simulink model "StateMachinaTesting"  (R2016a)
settings: Solver=VariableStepAuto  StartTime=0.0  StopTime=orbit_length*40  RelTol=1e-3
values from neighbouring files (symbols this model uses):
  A = eye(16,16)    [full_input_list.m]
  B = zeros(16,1)    [full_input_list.m]
  C = blkdiag(eye(3,3),zeros(3,3),eye(10,10))    [full_input_list.m]
  counter = 0    [full_input_list.m]
  deltaT = 0.00001    (= 1e-05)    [full_input_list.m]
  H = C    [full_input_list.m]
  kd = 0.5    [full_input_list.m]    (also in initACS.m = 0.01)
  kp = 1    [full_input_list.m]    (also in initACS.m = 0.01)
  OpModes = [0 0 0]    [full_input_list.m]
  OpTimes = [0 1 2]    [full_input_list.m]
  Q_k = zeros(16,16)    [full_input_list.m]
  R = R_k    [full_input_list.m]
  SeperationTime = 30000    [full_input_list.m]
  sim_start_time = (JD - JD_GPS0) * 24*60*60 - UTC_leap_seconds_wrt_GPS    (= 36000.0287935)    [full_input_list.m]
  st = 1/freq    (= 0.0125)    [full_input_list.m]    (also in initSimulink.m)
  u_k = zeros(16,1)    [full_input_list.m]
  w_k = zeros(16,1)    [full_input_list.m]
  x0 = [0 ... (first row only)    [full_input_list.m]
  Z_k = zeros(16,1)    [full_input_list.m]
undefined symbols (not defined in the file or in its folder): DiscIntNeverNeededParam, Earth, G_igrf, gyro_DCM_BS, H_igrf, I_undeployed, IAU, km, Kschmidt, mag_variance, n, R_mean, sat2, WGS84
libraries: simulink x29, dspmathops x24, aerolibutil x20, aerolibtransform2 x20, vrlib x15, aerolibgravity2 x5, dspinverses x4, SimMainLibrary x3, dspmtrx3 x1, lib_violet_env x1
(part 2 of 4)

== system StateMachinaTesting/Sensors MUXED/Center Cube Sensors ==
  note: TEMPORARY TO CHECK DATA EVALUATION AT LKF LEVEL
      | THIS IS AN ENTIRELY RBF SECTION
  note: r_N is in format:
      | - Lat (N-S) in decimal deg
      | - Long (E-W) in decimal deg
      | - Height in m
  State : Inport
  Add{1,3,5,7} (4 alike) : Sum
  Band-Limited White  Noise3 : simulink/Sources/Band-Limited White Noise  Cov=[1e-5]  Ts=0.1  seed=[23341]
  Band-Limited White Noise1 : simulink/Sources/Band-Limited White Noise  Cov=[0.1]  Ts=st  seed=[23341]
  Band-Limited White Noise5 : simulink/Sources/Band-Limited White Noise  Cov=[0.1]  Ts=0.1  seed=[23341]
  Band-Limited White Noise7 : simulink/Sources/Band-Limited White Noise  Cov=[0.1]  Ts=0.1  seed=[23341]
  Bus Creator2 : BusCreator  Inputs=6
  Bus Selector5 : BusSelector  OutputSignals=r_N,v_N,q_BN,w_BN
  Clock : Clock
  Constant : Constant  Value=sim_start_time
  Create Mag Vector : Subsystem
  Create Sun Vector : Subsystem  AncestorBlock=SimMainLibrary/SideCubeSensors/Create Sun Vector
  Derivative : Derivative
  Display : Display
  Subsystem : Subsystem
  Sum2 : Sum  Inputs=|++
  Sensors : Outport
  wires:
  Add1/1 -> Bus Creator2/1  "accelerometer_1"
  Band-Limited White Noise1/1 -> Add1/1
  Subsystem/1(a_B) -> Add1/2  "a_B"
  Band-Limited White  Noise3/1 -> Add3/1
  State/1 -> Bus Selector5/1
  Bus Creator2/1 -> Sensors/1
  Derivative/1 -> Subsystem/1("a_N ")  "a_N"
  Add7/1 -> Bus Creator2/3  "sun_B"
  Sum2/1 -> Create Sun Vector/2(time), Create Mag Vector/3(time), Bus Creator2/6  "time"
  Add3/1 -> Bus Creator2/2  "w_BN_1"
  Band-Limited White Noise7/1 -> Add7/1
  Create Sun Vector/1(sun_B) -> Add7/2  "sun_B"
  [r_N] -> Bus Creator2/4
  Create Mag Vector/1(mag_B) -> Add5/2
  Add5/1 -> Bus Creator2/5  "magnetometer_1"
  Band-Limited White Noise5/1 -> Add5/1
  [r_N] -> Create Mag Vector/2(r_N)
  Bus Selector5/1 -> [r_N]  "<r_N>"
  Bus Selector5/2 -> Derivative/1  "<v_N>"
  Bus Selector5/3 -> Subsystem/2(q_BN), Create Mag Vector/1(q_BN), Create Sun Vector/1(q_BN)  "<q_BN>"
  Bus Selector5/4 -> Add3/2  "<w_BN>"
  Constant/1 -> Sum2/1, Display/1
  Clock/1 -> Sum2/2

== system StateMachinaTesting/Sun Pointing/Target Quaternion ==
  w_c : Inport
  q4 : Inport  Port=2
  Constant : Constant  Value=pi
  Phi/2 : Trigonometry  Operator=acos
  Product : Product
  Terminator : Terminator
  Trigonometric Function1 : Trigonometry
  Trigonometric Function2 : Trigonometry  Operator=cos
  Vector Concatenate : Concatenate
  q_target : Outport
  wires:
  Vector Concatenate/1 -> q_target/1
  w_c/1 -> Product/1
  Product/1 -> Vector Concatenate/1
  Trigonometric Function1/1 -> Product/2
  Trigonometric Function2/1 -> Vector Concatenate/2
  q4/1 -> Phi/2/1
  Phi/2/1 -> Terminator/1
  Constant/1 -> Trigonometric Function2/1, Trigonometric Function1/1

== system StateMachinaTesting/x_measured1/Lookup Tables ==
  note: r_N is in format:
      | - Lat (N-S) in decimal deg
      | - Long (E-W) in decimal deg
      | - Height in m
  x_pos : Inport
  time : Inport  Port=2
  Demux : Demux  Outputs=3
  ECI Position to LLA : aerolibtransform2/ECI Position to LLA  Commented=on  red=IAU-2000/2006  year=2016  month=September  day=20  hour=0  min=0  sec=0  deltaT=Sec  errorflag=Error  extraparamflag=off  eunits=Metric (MKS)  earthmodel=WGS84  flat=1/298.257223563  eqradius=6378137
      settings: AttributesFormatString=%<red>
  GPS time to Jd sfrom J2000 : Subsystem
  Normalization : dspmathops/Normalization  NormType=2-norm  Bias=1e-10  NormOver=Each column  Dimension=1  outputDataTypeStr=Inherit: Same as product output  outputLastDataTypeStr=Inherit: Same as product output  outputMin=[]  outputMax=[]  accumDataTypeStr=Inherit: Same as product output  accumLastDataTypeStr=Inherit: Same as product output  roundingMode=Floor  overflowMode=off
  "RBF!!!!! " : Constant  Value=2015
  Sun position off of Jd frm J2000 : Subsystem
  Terminator{,1..3} (4 alike) : Terminator
  World Magnetic Model 2015 : aerolibgravity2/World Magnetic Model 2015  Commented=on  units=Metric (MKS)  time_in=on  month=January  day=1  year=2015  action=Error  h_out=on  dec_out=on  inc_out=on  ti_out=on
  B_N : Outport
  V_sun_N : Outport  Port=2
  wires:
  Sun position off of Jd frm J2000/1(Out1) -> Normalization/1
  GPS time to Jd sfrom J2000/1(Out1) -> Sun position off of Jd frm J2000/1(In1)
  Normalization/1 -> V_sun_N/1  "s_hat_N"
  time/1 -> ECI Position to LLA/2, GPS time to Jd sfrom J2000/1(In1)
  "RBF!!!!! "/1 -> World Magnetic Model 2015/4
  ECI Position to LLA/1 -> Demux/1
  x_pos/1 -> ECI Position to LLA/1
  World Magnetic Model 2015/5 -> Terminator3/1
  World Magnetic Model 2015/4 -> Terminator2/1
  World Magnetic Model 2015/3 -> Terminator1/1
  World Magnetic Model 2015/2 -> Terminator/1
  World Magnetic Model 2015/1 -> B_N/1
  Demux/2 -> World Magnetic Model 2015/3
  Demux/1 -> World Magnetic Model 2015/2
  Demux/3 -> World Magnetic Model 2015/1

== system StateMachinaTesting/x_measured1/q_N from Sensors ==
  B_B : Inport
  V_sun_B : Inport  Port=2
  B_N : Inport  Port=3
  V_sun_N : Inport  Port=4
  Cross Product{1..4} (4 alike) : vrlib/Utilities/Cross Product
  Direction Cosine Matrix to Quaternions : aerolibtransform2/Direction Cosine Matrix  to Quaternions
  Normalization{1..4} (4 alike) : dspmathops/Normalization  NormType=2-norm  Bias=1e-10  NormOver=Each column  Dimension=1  outputDataTypeStr=Inherit: Same as product output  outputLastDataTypeStr=Inherit: Same as product output  outputMin=[]  outputMax=[]  accumDataTypeStr=Inherit: Same as product output  accumLastDataTypeStr=Inherit: Same as product output  roundingMode=Floor  overflowMode=off
  Product : Product  Multiplication=Matrix(*)
  Pseudoinverse : dspinverses/Pseudoinverse  wanterr=off
  Vector Concatenate : Concatenate  NumInputs=3  Mode=Multidimensional array  ConcatenateDimension=2
  Vector Concatenate1 : Concatenate  NumInputs=3  Mode=Multidimensional array  ConcatenateDimension=2
  quat From DCM : MATLAB Function  Commented=on  TreatAsAtomicUnit=on
  q_N : Outport
  Q : Outport  Port=2
  wires:
  Vector Concatenate1/1 -> Pseudoinverse/1
  Pseudoinverse/1 -> Product/2
  Product/1 -> Q/1, Direction Cosine Matrix to Quaternions/1
  Vector Concatenate/1 -> Product/1
  Cross Product4/1 -> Vector Concatenate/1  "n_1"
  Normalization3/1 -> Cross Product4/2, Vector Concatenate/3  "n_3"
  Normalization4/1 -> Cross Product4/1, Vector Concatenate/2  "n_2"
  Cross Product2/1 -> Normalization3/1
  B_N/1 -> Normalization4/1, Cross Product2/2
  Cross Product3/1 -> Vector Concatenate1/1  "b_1"
  Normalization1/1 -> Cross Product3/2, Vector Concatenate1/3  "b_3"
  Normalization2/1 -> Cross Product3/1, Vector Concatenate1/2  "b_2"
  Cross Product1/1 -> Normalization1/1
  B_B/1 -> Normalization2/1, Cross Product1/2
  V_sun_B/1 -> Cross Product1/1
  V_sun_N/1 -> Cross Product2/1
  Direction Cosine Matrix to Quaternions/1 -> q_N/1

== system StateMachinaTesting/Flight Controller/Center Cube Controller/Attitude Compensator ==
  note: Commands of 4 burn wires; two for sidecube deploy
      | and two for stabilizing wires
  note: Action Block
      | Notes: This block determines the actions the satellite will execute based on the commands given by ground control/ powerboard.
      | -Possible we end up combining this and the guidance block for simplicity
  SafedOpMode : Inport
  SafedSepBurn : Inport  Port=2
  q2 : Inport  Port=3
  w2 : Inport  Port=4
  Bus Creator : BusCreator  Inputs=2
  Constant : Constant  Value=[ 1 1 1 1 ]
  Deployed Modes (switch)1 : Subsystem
  Merge2 : Merge
  Not Deployed Modes (switch) : Subsystem
  Selector : Selector  InputPortWidth=4  IndexOptions=Index vector (dialog)  Indices=[1]  OutputSizes=1
  Switch Case : SwitchCase  CaseConditions={0,1}  ShowDefaultCase=off
  Terminator : Terminator
  OpMode : Outport
  SepBurn : Outport  Port=2
  Tau1 : Outport  Port=3
  wires:
  SafedOpMode/1 -> [OpMode], OpMode/1
  Merge2/1 -> Tau1/1
  Not Deployed Modes (switch)/1(Out1) -> Merge2/1
  q2/1 -> [Quaternion]
  w2/1 -> [SpinRate]
  [Quaternion] -> Not Deployed Modes (switch)/2(q_BN)
  [SpinRate] -> Not Deployed Modes (switch)/3(w_BN)
  [Quaternion] -> Deployed Modes (switch)1/2(q1)
  [SpinRate] -> Deployed Modes (switch)1/3(w1)
  Deployed Modes (switch)1/1(Out1) -> Merge2/2
  [SafedSepBurn] -> Selector/1
  Constant/1 -> SepBurn/1, [SafedSepBurn]
  Switch Case/1 -> Not Deployed Modes (switch)/Action  "SafedSepBurn"
  Switch Case/2 -> Deployed Modes (switch)1/Action  "SafedSepBurn"
  [OpMode] -> Bus Creator/1
  Bus Creator/1 -> Not Deployed Modes (switch)/1(Mode and BurnCmd), Deployed Modes (switch)1/1(Mode and BurnCmd)
  [SafedSepBurn] -> Bus Creator/2  "SeperationCommand"
  SafedSepBurn/1 -> Terminator/1
  Selector/1 -> Switch Case/1

== system StateMachinaTesting/Flight Controller/Center Cube Controller/Motor Control Placeholder ==
  note: Tether Control Sybsystem
      | When the spin rate of the CubeSat reaches
      | 6rpm, the tether will unreel a set amount
  spin rate : Inport
  SafedOpMode : Inport  Port=2
  If : If  NumInputs=2  IfExpression=u1 > 5 & u2 > 0
  Math Function : Math  Operator=square  SaturateOnIntegerOverflow=on
  Merge : Merge
  Mux : Mux  Inputs=2
  Spinning fast : Subsystem  TreatAsAtomicUnit=on
  Spinning slow : Subsystem  TreatAsAtomicUnit=on
  Sqrt : Sqrt  SaturateOnIntegerOverflow=on
  Sum of Elements : Sum  Inputs=+
  motor cmd : Outport
  wires:
  Math Function/1 -> Sum of Elements/1
  Sum of Elements/1 -> Sqrt/1
  spin rate/1 -> Math Function/1
  Sqrt/1 -> If/1
  Spinning fast/1(Out1) -> Merge/1
  Spinning slow/1(Out1) -> Merge/2
  If/1 -> Spinning fast/Action
  If/2 -> Spinning slow/Action
  SafedOpMode/1 -> If/2
  Mux/1 -> motor cmd/1
  Merge/1 -> Mux/2, Mux/1

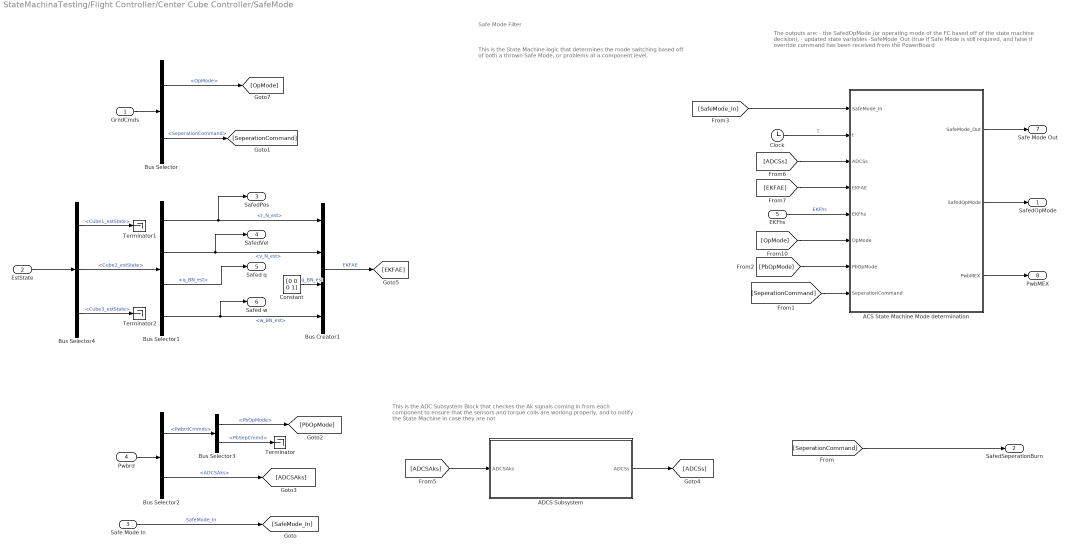
== system StateMachinaTesting/Flight Controller/Center Cube Controller/SafeMode ==
  note: This is the State Machine logic that determines the mode switching based off of both a thrown Safe Mode, or problems at a component level.
  note: Safe Mode Filter
  note: The outputs are:
      | - the SafedOpMode (or operating mode of the FC based off of the state machine decision),
      | - updated state variables
      | -SafeMode_Out (true if Safe Mode is still required, and false if override command has been received from the PowerBoard
  note: This is the ADC Subsystem Block that checkes the Ak signals coming in from each component to ensure that the sensors and torque coils are working properly, and to notify the State Machine in case they are not
  GrndCmds : Inport
  EstState : Inport  Port=2
  Safe Mode In : Inport  Port=3
  Pwbrd : Inport  Port=4
  "EKFhs " : Inport  Port=5
  ACS State Machine Mode determination : MATLAB Function  TreatAsAtomicUnit=on
  ADCS Subsystem : Subsystem
  Bus Creator1 : BusCreator  Inputs='r_N_est','v_N_est','q_BN_est','w_BN_est'
  Bus Selector : BusSelector  OutputSignals=OpMode,SeperationCommand
  Bus Selector1 : BusSelector  OutputSignals=r_N_est,v_N_est,q_BN_est,w_BN_est
  Bus Selector2 : BusSelector  OutputSignals=PwbrdCmmds,ADCSAks
  Bus Selector3 : BusSelector  OutputSignals=PbOpMode,PbSepCmmd
  Bus Selector4 : BusSelector  OutputSignals=Cube1_estState,Cube2_estState,Cube3_estState
  Clock : Clock
  Constant : Constant  Value=[0 0 0 1]
  Terminator : Terminator
  Terminator1 : Terminator
  Terminator2 : Terminator
  SafedOpMode : Outport
  SafedSeperationBurn : Outport  Port=2
  SafedPos : Outport  Port=3
  SafedVel : Outport  Port=4
  Safed q : Outport  Port=5
  Safed w : Outport  Port=6
  Safe Mode Out : Outport  Port=7
  PwbMEX : Outport  Port=8
  wires:
  Clock/1 -> ACS State Machine Mode determination/2(t)  "t"
  "EKFhs "/1 -> ACS State Machine Mode determination/5(EKFhs)  "EKFhs"
  [ADCSs] -> ACS State Machine Mode determination/3(ADCSs)
  Bus Selector1/4 -> Safed w/1, Bus Creator1/4  "<w_BN_est>"
  Bus Selector1/3 -> Safed q/1  "<q_BN_est>"
  Bus Selector1/2 -> SafedVel/1, Bus Creator1/2  "<v_N_est>"
  Bus Selector1/1 -> SafedPos/1, Bus Creator1/1  "<r_N_est>"
  EstState/1 -> Bus Selector4/1
  Bus Selector/1 -> [OpMode]  "<OpMode>"
  GrndCmds/1 -> Bus Selector/1
  Safe Mode In/1 -> [SafeMode_In]  "SafeMode_In"
  ACS State Machine Mode determination/1(SafeMode_Out) -> Safe Mode Out/1
  Bus Selector/2 -> [SeperationCommand]  "<SeperationCommand>"
  [SeperationCommand] -> SafedSeperationBurn/1
  [SeperationCommand] -> ACS State Machine Mode determination/8(SeperationCommand)
  Pwbrd/1 -> Bus Selector2/1
  Bus Selector2/2 -> [ADCSAks]  "<ADCSAks>"
  [ADCSAks] -> ADCS Subsystem/1("ADCSAks ")
  Bus Selector2/1 -> Bus Selector3/1  "<PwbrdCmmds>"
  Bus Selector3/1 -> [PbOpMode]  "<PbOpMode>"
  [OpMode] -> ACS State Machine Mode determination/6(OpMode)
  [PbOpMode] -> ACS State Machine Mode determination/7(PbOpMode)
  Bus Creator1/1 -> [EKFAE]  "EKFAE"
  [EKFAE] -> ACS State Machine Mode determination/4(EKFAE)
  ACS State Machine Mode determination/2(SafedOpMode) -> SafedOpMode/1
  ACS State Machine Mode determination/3(PwbMEX) -> PwbMEX/1
  Bus Selector3/2 -> Terminator/1  "<PbSepCmmd>"
  ADCS Subsystem/1("ADCSs ") -> [ADCSs]
  [SafeMode_In] -> ACS State Machine Mode determination/1(SafeMode_In)
  Constant/1 -> Bus Creator1/3  "q_BN_est"
  Bus Selector4/2 -> Bus Selector1/1  "<Cube2_estState>"
  Bus Selector4/1 -> Terminator1/1  "<Cube1_estState>"
  Bus Selector4/3 -> Terminator2/1  "<Cube3_estState>"

== system StateMachinaTesting/Flight Controller/Center Cube Controller/Torque Coil Management ==
  note: Navigation Block
      | This block takes in data from the Actions/guidance block as to the current attitude of the spacecraft, the desired attitude of the spacecraft, and the required torque and outputs the current necessary to be applied to the torque coils as well as the torque currently being applied by the torque coils.
  BurnCmd : Inport
  q_BN : Inport  Port=2
  w : Inport  Port=3
  tau_B : Inport  Port=4
  b_N : Inport  Port=5
  Clock : Clock
  Constant : Constant
  Constant b_N field RBF!!!!!!!!!!!!!!!! SUB IN THE b_N : Constant  Value=[1 1 1]
  Constant1 : Constant
  Counter : Constant  Value=counter
  If : If  NumInputs=2  IfExpression=(u1 > 0)|(u2>5)
  Measurement Predicition : Subsystem
  Merge1 : Merge
  Merge2 : Merge
  No Action : Subsystem  TreatAsAtomicUnit=on
  PD Controller : Subsystem
  Selector : Selector  Commented=on  InputPortWidth=4  IndexOptions=Index vector (dialog)  Indices=[1]  OutputSizes=1
  Terminator : Terminator
  Terminator1 : Terminator
  Terminator3 : Terminator
  Torque Coil Management : Subsystem  TreatAsAtomicUnit=on
  CenterCube_PWM_cmds : Outport
  torque_coils : Outport  Port=2
  wires:
  BurnCmd/1 -> Selector/1
  If/1 -> Torque Coil Management/Action
  Merge1/1 -> CenterCube_PWM_cmds/1
  Merge2/1 -> torque_coils/1
  Torque Coil Management/1(current_coils) -> Merge1/1
  Torque Coil Management/2(torque_coils) -> Merge2/1
  No Action/1(I_coils) -> Merge1/2
  No Action/2(torque_coils) -> Merge2/2
  q_BN/1 -> Torque Coil Management/2(q_BN)
  tau_B/1 -> Torque Coil Management/1(tau_B)
  w/1 -> PD Controller/1(In1)
  PD Controller/1(torque_coils) -> Terminator3/1
  Measurement Predicition/1(predicition) -> Terminator1/1
  Clock/1 -> Torque Coil Management/4(t)
  If/2 -> No Action/Action
  Counter/1 -> If/2
  Constant/1 -> Measurement Predicition/1(GPS_time)
  Constant1/1 -> Measurement Predicition/2(something else)
  Selector/1 -> If/1
  Constant b_N field RBF!!!!!!!!!!!!!!!! SUB IN THE b_N/1 -> Torque Coil Management/3(b_N)
  b_N/1 -> Terminator/1

== system StateMachinaTesting/Flight Controller/CenterCube EKF/Kalman Gain and Estamated State Computation ==
  P_kp : Inport
  x_kp : Inport  Port=2
  Y : Inport  Port=3
  " LU Inverse" : dspinverses/ LU Inverse
  Add1 : Sum
  Add2 : Sum
  Add3 : Sum  Inputs=-+
  H : Constant  Value=H
  H1 : Constant  Value=H
  Math Function : Math  Operator=transpose  SaturateOnIntegerOverflow=on
  Product{,1,3..4,6} (5 alike) : Product  Multiplication=Matrix(*)
  Product2 : Product
  R : Constant  Value=R
  K : Outport
  x_k : Outport  Port=2
  wires:
  H/1 -> Product3/1, Product1/2, Math Function/1
  " LU Inverse"/1 -> Product/2
  Product1/1 -> Product/1
  Math Function/1 -> Product4/2
  Product/1 -> Product2/1, K/1  "Kalman Gain K"
  x_kp/1 -> Add2/1, Product6/2
  Y/1 -> Add3/2
  R/1 -> Add1/2
  Product4/1 -> Add1/1
  Add1/1 -> " LU Inverse"/1
  Product3/1 -> Product4/1
  H1/1 -> Product6/1
  Product6/1 -> Add3/1
  P_kp/1 -> Product3/2, Product1/1
  Add2/1 -> x_k/1
  Add3/1 -> Product2/2
  Product2/1 -> Add2/2

== system StateMachinaTesting/Flight Controller/CenterCube EKF/New State Prediction  ==
  note: LKF
  note: EKF
  P_k-1 : Inport
  x_k-1 : Inport  Port=2
  A_LKF : Subsystem
  Add1 : Sum  Inputs=+++
  Add2 : Sum
  Add3 : Sum
  B : Constant  Value=B
  Math Function : Math  Operator=transpose  SaturateOnIntegerOverflow=on
  Math Function1 : Math  Operator=transpose  SaturateOnIntegerOverflow=on
  Predictions : MATLAB Function  TreatAsAtomicUnit=on
  Product{,1..5} (6 alike) : Product  Multiplication=Matrix(*)
  Q_k : Constant  Value=Q_k
  Q_k1 : Constant  Value=Q_k
  Terminator2 : Terminator
  Terminator3 : Terminator
  u_k : Constant  Value=u_k
  w_k : Constant  Value=w_k
  P_kp : Outport
  "x_kp  " : Outport  Port=2
  wires:
  Product2/1 -> Product3/1
  Math Function/1 -> Product3/2
  Product/1 -> Add1/1
  B/1 -> Product1/1
  Product1/1 -> Add1/2
  u_k/1 -> Product1/2
  w_k/1 -> Add1/3
  Q_k/1 -> Add2/2
  P_k-1/1 -> [A], Product2/2
  Product3/1 -> Add2/1
  x_k-1/1 -> Predictions/1(x_ko), Product/2, A_LKF/1(In1)
  A_LKF/1(Out1) -> Product2/1, Math Function/1, Product/1  "A"
  Predictions/1(F) -> Math Function1/1, Product4/1
  [A] -> Product4/2
  Product4/1 -> Product5/1
  Math Function1/1 -> Product5/2
  Predictions/2(x_kp) -> "x_kp  "/1  "x_kps"
  Product5/1 -> Add3/1
  Q_k1/1 -> Add3/2
  Add3/1 -> P_kp/1  "P_kp"
  Add2/1 -> Terminator2/1  "P_kp"
  Add1/1 -> Terminator3/1  "x_kp"

== system StateMachinaTesting/Flight Controller/CenterCube EKF/Y computation ==
  In1 : Inport
  Add2 : Sum
  C : Constant  Value=C
  Product2 : Product  Multiplication=Matrix(*)
  "Z_k " : Constant  Value=Z_k
  Y : Outport
  wires:
  Add2/1 -> Y/1
  "Z_k "/1 -> Add2/2
  In1/1 -> Product2/2
  C/1 -> Product2/1
  Product2/1 -> Add2/1

== system StateMachinaTesting/Flight Controller/CenterCube EKF/x_measured ==
  Sensor_data : Inport
  Bus Selector1 : BusSelector  OutputSignals=w_BN_1,magnetometer_1,sun_B,r_N,accelerometer_1,time
  Constant : Constant  Value=[0;0;0]
  Lookup Tables : Subsystem
  Terminator : Terminator
  Vector Concatenate : Concatenate  NumInputs=5
  q_N from Sensors : Subsystem
  x_measured : Outport
  B_N : Outport  Port=2
  wires:
  Bus Selector1/4 -> Vector Concatenate/1, Lookup Tables/1(x_pos)  "<r_N>"
  Vector Concatenate/1 -> x_measured/1
  Lookup Tables/2(V_sun_N) -> q_N from Sensors/4(V_sun_N)
  Bus Selector1/3 -> q_N from Sensors/2(V_sun_B)  "<sun_B>"
  Lookup Tables/1(B_N) -> B_N/1, q_N from Sensors/3(B_N)
  q_N from Sensors/2(Q) -> Terminator/1
  Sensor_data/1 -> Bus Selector1/1
  Bus Selector1/1 -> Vector Concatenate/4  "<w_BN_1>"
  Constant/1 -> Vector Concatenate/2  "xdot_measured"
  Bus Selector1/5 -> Vector Concatenate/3  "<accelerometer_1>"
  q_N from Sensors/1(q_N) -> Vector Concatenate/5  "quat_measured"
  Bus Selector1/2 -> q_N from Sensors/1(B_B)  "<magnetometer_1>"
  Bus Selector1/6 -> Lookup Tables/2(time)  "<time>"

== system StateMachinaTesting/Flight Controller/CenterCube EKF/x_measured1 ==
  Sensor_data : Inport
  Bus Selector1 : BusSelector  OutputSignals=w_BN_1,magnetometer_1,sun_B,r_N,accelerometer_1,time
  Lookup Tables : Subsystem
  Name change : MATLAB Function  TreatAsAtomicUnit=on
  Name change1 : MATLAB Function  TreatAsAtomicUnit=on
  Terminator : Terminator
  Terminator1 : Terminator
  q_N from Sensors : Subsystem
  vis viva : MATLAB Function  TreatAsAtomicUnit=on
  r_N_est : Outport
  v_N_est : Outport  Port=2
  w_BN_est : Outport  Port=3
  q_BN_est : Outport  Port=4
  wires:
  Bus Selector1/6 -> Lookup Tables/2(time)  "<time>"
  Bus Selector1/2 -> q_N from Sensors/1(B_B)  "<magnetometer_1>"
  q_N from Sensors/1(q_N) -> q_BN_est/1  "q_BN_est"
  Sensor_data/1 -> Bus Selector1/1
  q_N from Sensors/2(Q) -> Terminator/1
  Lookup Tables/1(B_N) -> q_N from Sensors/3(B_N)
  Bus Selector1/3 -> q_N from Sensors/2(V_sun_B)  "<sun_B>"
  Lookup Tables/2(V_sun_N) -> q_N from Sensors/4(V_sun_N)
  Bus Selector1/4 -> Name change/1(u), Lookup Tables/1(x_pos)  "<r_N>"
  Name change1/1(y) -> w_BN_est/1  "w_BN_est"
  Bus Selector1/1 -> Name change1/1(u)  "<w_BN_1>"
  Bus Selector1/5 -> Terminator1/1  "<accelerometer_1>"
  Name change/1(y) -> r_N_est/1, vis viva/1(x)  "r_N_est"
  vis viva/1(xdot) -> v_N_est/1  "v_N_est"

== system StateMachinaTesting/Inital Spin Up/Target Quaternion/Aligned ==
  q4 : Inport
  t_curr : Inport  Port=2
  t_old : Inport  Port=3
  Action Port : ActionPort  ActionType=then
  Gain : Gain  Gain=1/2
  Phi : Gain  Gain=2
  Phi+dPhi : Sum
  Phi/2 : Trigonometry  Operator=acos
  Subsystem : Subsystem
  Phi/2_new : Outport
  wires:
  q4/1 -> Phi/2/1
  Phi/2/1 -> Phi/1
  Phi+dPhi/1 -> Gain/1
  t_curr/1 -> Subsystem/1(t_curr)
  Phi/1 -> Phi+dPhi/2
  Gain/1 -> Phi/2_new/1
  Subsystem/1(dPhi) -> Phi+dPhi/1
  t_old/1 -> Subsystem/2(t_old)

== system StateMachinaTesting/Inital Spin Up/Target Quaternion/Aligned1 ==
  q4 : Inport
  t_curr : Inport  Port=2
  t_old : Inport  Port=3
  Action Port : ActionPort  ActionType=else
  Gain : Gain  Gain=1/2
  Phi : Gain  Gain=2
  Phi+dPhi : Sum
  Phi/2 : Trigonometry  Operator=acos
  Subsystem : Subsystem
  Phi/2_new : Outport
  wires:
  q4/1 -> Phi/2/1
  Phi/2/1 -> Phi/1
  Phi+dPhi/1 -> Gain/1
  t_curr/1 -> Subsystem/1(t_curr)
  Phi/1 -> Phi+dPhi/2
  Gain/1 -> Phi/2_new/1
  Subsystem/1(dPhi) -> Phi+dPhi/1
  t_old/1 -> Subsystem/2(t_old)

== system StateMachinaTesting/Inital Spin Up/Target Quaternion/Not Aligned ==
  q4 : Inport
  Action Port : ActionPort
  Constant : Constant  Value=pi
  Phi/2 : Trigonometry  Operator=acos
  Terminator : Terminator
  Phi/2_new : Outport
  wires:
  q4/1 -> Phi/2/1
  Phi/2/1 -> Phi/2_new/1
  Constant/1 -> Terminator/1

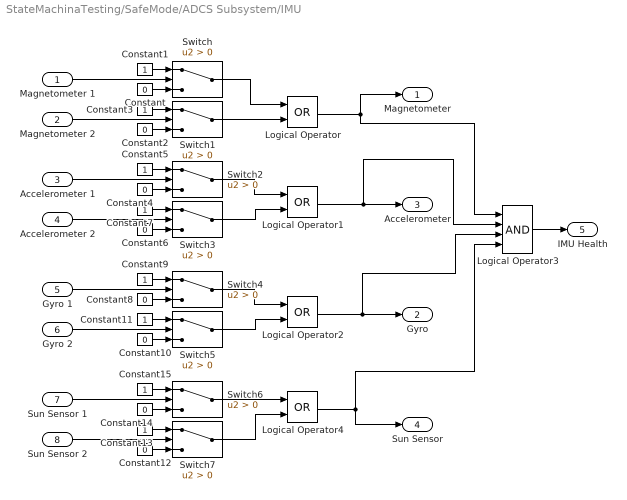
== system StateMachinaTesting/SafeMode/ADCS Subsystem/IMU ==
  Magnetometer 1 : Inport
  Magnetometer 2 : Inport  Port=2
  Accelerometer 1 : Inport  Port=3
  " Accelerometer 2" : Inport  Port=4
  Gyro 1 : Inport  Port=5
  Gyro 2 : Inport  Port=6
  Sun Sensor 1 : Inport  Port=7
  Sun Sensor 2 : Inport  Port=8
  Constant{,2,4,6,8,10,12,14} (8 alike) : Constant  Value=0
  Constant{1,3,5,7,9,11,13,15} (8 alike) : Constant
  Logical Operator{,1..2,4} (4 alike) : Logic  Operator=OR  AllPortsSameDT=off  OutDataTypeStr=boolean
  Logical Operator3 : Logic  Inputs=4  AllPortsSameDT=off  OutDataTypeStr=boolean
  Switch{,1..7} (8 alike) : Switch  Criteria=u2 > Threshold
  Magnetometer : Outport
  "Gyro " : Outport  Port=2
  Accelerometer : Outport  Port=3
  "Sun Sensor " : Outport  Port=4
  IMU Health : Outport  Port=5
  wires:
  Logical Operator3/1 -> IMU Health/1
  Switch7/1 -> Logical Operator4/2
  Constant12/1 -> Switch7/3
  Constant13/1 -> Switch7/1
  Switch6/1 -> Logical Operator4/1
  Constant14/1 -> Switch6/3
  Constant15/1 -> Switch6/1
  Logical Operator4/1 -> Logical Operator3/4, "Sun Sensor "/1
  Switch5/1 -> Logical Operator2/2
  Constant10/1 -> Switch5/3
  Constant11/1 -> Switch5/1
  Switch4/1 -> Logical Operator2/1
  Constant8/1 -> Switch4/3
  Constant9/1 -> Switch4/1
  Switch3/1 -> Logical Operator1/2
  Constant6/1 -> Switch3/3
  Constant7/1 -> Switch3/1
  Switch2/1 -> Logical Operator1/1
  Constant4/1 -> Switch2/3
  Constant5/1 -> Switch2/1
  Switch1/1 -> Logical Operator/2
  Constant2/1 -> Switch1/3
  Constant3/1 -> Switch1/1
  Switch/1 -> Logical Operator/1
  Constant/1 -> Switch/3
  Constant1/1 -> Switch/1
  Magnetometer 1/1 -> Switch/2
  Logical Operator2/1 -> "Gyro "/1, Logical Operator3/3
  Logical Operator1/1 -> Accelerometer/1, Logical Operator3/2
  Logical Operator/1 -> Logical Operator3/1, Magnetometer/1
  Magnetometer 2/1 -> Switch1/2
  Gyro 1/1 -> Switch4/2
  Gyro 2/1 -> Switch5/2
  Sun Sensor 1/1 -> Switch6/2
  Sun Sensor 2/1 -> Switch7/2
  " Accelerometer 2"/1 -> Switch3/2
  Accelerometer 1/1 -> Switch2/2

== system StateMachinaTesting/SafeMode/ADCS Subsystem/Magnetic Torquers ==
  Magnetorquer X1 : Inport
  Magnetometer Y1 : Inport  Port=2
  Magnetometer Z1 : Inport  Port=3
  Constant : Constant  Value=0
  Constant1 : Constant
  Constant4 : Constant  Value=0
  Constant5 : Constant
  Constant8 : Constant  Value=0
  Constant9 : Constant
  Logical Operator3 : Logic  Inputs=3  AllPortsSameDT=off  OutDataTypeStr=boolean
  Switch : Switch  Criteria=u2 > Threshold
  Switch2 : Switch  Criteria=u2 > Threshold
  Switch4 : Switch  Criteria=u2 > Threshold
  X Torquer Status : Outport
  "Y Torquer Status " : Outport  Port=2
  Z Torquer Status : Outport  Port=3
  Actuator Health : Outport  Port=4
  wires:
  Logical Operator3/1 -> Actuator Health/1
  Constant8/1 -> Switch4/3
  Constant9/1 -> Switch4/1
  Magnetometer Z1/1 -> Switch4/2
  Constant4/1 -> Switch2/3
  Constant5/1 -> Switch2/1
  Magnetometer Y1/1 -> Switch2/2
  Constant/1 -> Switch/3
  Constant1/1 -> Switch/1
  Magnetorquer X1/1 -> Switch/2
  Switch4/1 -> Z Torquer Status/1, Logical Operator3/3
  Switch2/1 -> "Y Torquer Status "/1, Logical Operator3/2
  Switch/1 -> X Torquer Status/1, Logical Operator3/1

== system StateMachinaTesting/Sensors BUSSED/Center Cube Sensors/Create Mag Vector ==
  q_BN : Inport
  r_N : Inport  Port=2
  Constant : Constant  Value=[1 1 1]
  Terminator : Terminator
  Terminator1 : Terminator
  mag_B : Outport
  wires:
  Constant/1 -> mag_B/1
  r_N/1 -> Terminator1/1
  q_BN/1 -> Terminator/1

== system StateMachinaTesting/Sensors BUSSED/Center Cube Sensors/Create Mag Vector1 ==
  note: r_N is in format:
      | - Lat (N-S) in decimal deg
      | - Long (E-W) in decimal deg
      | - Height in m
  q_BN : Inport
  r_N : Inport  Port=2
  time : Inport  Port=3
  Constant : Constant  Value=1e-9
  Demux : Demux  Outputs=3
  ECI Position to LLA : aerolibtransform2/ECI Position to LLA  red=IAU-2000/2006  year=2016  month=September  day=20  hour=0  min=0  sec=0  deltaT=Sec  errorflag=Error  extraparamflag=off  eunits=Metric (MKS)  earthmodel=WGS84  flat=1/298.257223563  eqradius=6378137
      settings: AttributesFormatString=%<red>
  Product : Product  Multiplication=Matrix(*)
  Product1 : Product
  Quaternions to Direction Cosine Matrix : aerolibtransform2/Quaternions to  Direction Cosine Matrix
  "RBF!!!!! " : Constant  Value=2015
  Terminator{2..5} (4 alike) : Terminator
  World Magnetic Model 2015 : aerolibgravity2/World Magnetic Model 2015  units=Metric (MKS)  time_in=on  month=January  day=1  year=2015  action=Error  h_out=on  dec_out=on  inc_out=on  ti_out=on
  mag_B : Outport
  wires:
  Product/1 -> mag_B/1
  Demux/1 -> World Magnetic Model 2015/2
  Demux/2 -> World Magnetic Model 2015/3
  World Magnetic Model 2015/2 -> Terminator2/1
  World Magnetic Model 2015/3 -> Terminator3/1
  World Magnetic Model 2015/4 -> Terminator4/1
  World Magnetic Model 2015/5 -> Terminator5/1
  time/1 -> ECI Position to LLA/2
  "RBF!!!!! "/1 -> World Magnetic Model 2015/4
  r_N/1 -> ECI Position to LLA/1
  Demux/3 -> World Magnetic Model 2015/1
  ECI Position to LLA/1 -> Demux/1
  q_BN/1 -> Quaternions to Direction Cosine Matrix/1
  Quaternions to Direction Cosine Matrix/1 -> Product/1
  World Magnetic Model 2015/1 -> Product1/2
  Constant/1 -> Product1/1
  Product1/1 -> Product/2

== system StateMachinaTesting/Sensors BUSSED/Center Cube Sensors/Create Sun Vector ==
  note: s_hat_N
  note: Outputs the unit vector towards the sun wrt the body (or earth; doesn't matter) in the inertial frame (N).
  q_BN : Inport
  GPS time : Inport  Port=2
  GPS time to Jd sfrom J2000 : Subsystem
  Normalization : dspmathops/Normalization  NormType=2-norm  Bias=1e-10  NormOver=Each column  Dimension=1  outputDataTypeStr=Inherit: Same as product output  outputLastDataTypeStr=Inherit: Same as product output  outputMin=[]  outputMax=[]  accumDataTypeStr=Inherit: Same as product output  accumLastDataTypeStr=Inherit: Same as product output  roundingMode=Floor  overflowMode=off
  Product : Product  Multiplication=Matrix(*)
  Quaternions to Direction Cosine Matrix : aerolibtransform2/Quaternions to  Direction Cosine Matrix
  Sun position off of Jd frm J2000 : Subsystem
  sun_B : Outport
  wires:
  GPS time/1 -> GPS time to Jd sfrom J2000/1(In1)
  Product/1 -> sun_B/1
  q_BN/1 -> Quaternions to Direction Cosine Matrix/1
  Normalization/1 -> Product/2
  Quaternions to Direction Cosine Matrix/1 -> Product/1
  GPS time to Jd sfrom J2000/1(Out1) -> Sun position off of Jd frm J2000/1(In1)
  Sun position off of Jd frm J2000/1(Out1) -> Normalization/1

== system StateMachinaTesting/Sensors BUSSED/Center Cube Sensors/Create Sun Vector1 ==
  note: s_hat_N
  note: Outputs the unit vector towards the sun wrt the body (or earth; doesn't matter) in the inertial frame (N).
  q_BN : Inport
  time : Inport  Port=2
  GPS time to Jd sfrom J2000 : Subsystem
  Normalization : dspmathops/Normalization  NormType=2-norm  Bias=1e-10  NormOver=Each column  Dimension=1  outputDataTypeStr=Inherit: Same as product output  outputLastDataTypeStr=Inherit: Same as product output  outputMin=[]  outputMax=[]  accumDataTypeStr=Inherit: Same as product output  accumLastDataTypeStr=Inherit: Same as product output  roundingMode=Floor  overflowMode=off
  Product : Product  Multiplication=Matrix(*)
  Quaternions to Direction Cosine Matrix : aerolibtransform2/Quaternions to  Direction Cosine Matrix
  Sun position off of Jd frm J2000 : Subsystem
  sun_B : Outport
  wires:
  time/1 -> GPS time to Jd sfrom J2000/1(In1)
  Product/1 -> sun_B/1
  q_BN/1 -> Quaternions to Direction Cosine Matrix/1
  Normalization/1 -> Product/2
  Quaternions to Direction Cosine Matrix/1 -> Product/1
  GPS time to Jd sfrom J2000/1(Out1) -> Sun position off of Jd frm J2000/1(In1)
  Sun position off of Jd frm J2000/1(Out1) -> Normalization/1

== system StateMachinaTesting/Sensors BUSSED/Center Cube Sensors/GPS ==
  note: Position in the sensor reference frame
  note: GPS Sensor Spoofing
      | We must specify the GPS variance and seed later when we have more time
      |
      | DCM of ECFE wrt ECI is not filled in
      |
      | GPS start time needs to be filled in.
      |
      | Violet was able to check for corrupt signals - that is the next step
  note: Velocity in the sensor reference frame
  r_N : Inport
  v_N : Inport  Port=2
  DCM of ECFC wrt ECI : Constant  Value=eye(3)
  DCM of ECFC wrt ECI1 : Constant  Value=eye(3)
  Digital Clock : DigitalClock
  GPS start time : Constant  Value=0
  Position random noise : RandomNumber  SampleTime=0.1
  Product : Product
  Product1 : Product
  Sum : Sum
  Sum1 : Sum
  Sum2 : Sum  Inputs=|++
  Velocity random noise : RandomNumber  SampleTime=0.1
  r_S : Outport
  v_S : Outport  Port=2
  Time : Outport  Port=3
  wires:
  Sum/1 -> r_S/1
  Position random noise/1 -> Sum/2
  Sum1/1 -> v_S/1
  Velocity random noise/1 -> Sum1/2
  GPS start time/1 -> Sum2/1
  Digital Clock/1 -> Sum2/2
  Sum2/1 -> Time/1
  DCM of ECFC wrt ECI/1 -> Product/1
  r_N/1 -> Product/2
  Product/1 -> Sum/1
  DCM of ECFC wrt ECI1/1 -> Product1/1
  v_N/1 -> Product1/2
  Product1/1 -> Sum1/1

== system StateMachinaTesting/Sensors BUSSED/Center Cube Sensors/Gyro ==
  note: Gyro Sensor Spoofing
      |
      | Lots of work left to be done on the Gyro. Violet tracks the gyro bias - necessary?
      |
      | Violet also records the time of the gyro - is this simply a diagnostic step?
  w_BN_B : Inport
  Bias : MATLAB Function  TreatAsAtomicUnit=on
  Bus Creator : BusCreator  Inputs=2
  Digital Clock : DigitalClock
  Discrete-Time Integrator : DiscreteIntegrator  gainval=1  InitialConditionSetting=State (most efficient)  ICPrevOutput=DiscIntNeverNeededParam  ICPrevScaledInput=DiscIntNeverNeededParam
  Gyro_DCM_BS : Constant  Value=gyro_DCM_BS
  Product : Product  Multiplication=Matrix(*)
  Random Bias Steps : RandomNumber  SampleTime=0.1
  Random Noise : RandomNumber  SampleTime=0.1
  Sum : Sum
  w_SN_S_m : Outport
  time : Outport  Port=2
  Gyro : Outport  Port=3
  wires:
  w_BN_B/1 -> Product/2
  Random Bias Steps/1 -> Discrete-Time Integrator/1
  Product/1 -> Sum/1
  Discrete-Time Integrator/1 -> Sum/2
  Sum/1 -> Bias/1(w)
  Random Noise/1 -> Bias/2(noise)
  Bias/1(wn) -> Bus Creator/1, w_SN_S_m/1
  Gyro_DCM_BS/1 -> Product/1
  Digital Clock/1 -> Bus Creator/2, time/1
  Bus Creator/1 -> Gyro/1

== system StateMachinaTesting/Sensors BUSSED/Center Cube Sensors/Magnetometer ==
  note: Teslas to Gauss
  note: from r_E to b_B is in Violet Dynamics Block.
      | The rest is in their sensor block.
  note: b_B
  note: DCM of Body wrt Neutral
  note: Pulled from NASA Langley
  note: The block takes the magnetic field in the body reference frame
      | and transforms it into magnetic field in the sensor reference
      | frame.
      |
      | We still need the DCM and the variance of the magnetometer
  r_E : Inport  PortDimensions=[1 3]
  Bus Creator : BusCreator  Inputs=2
  DCM B wrt S : Constant  Value=eye(3)
  DCM of BN : Constant  Value=eye(3)
  DCM of ECFC wrt ECI : Constant  Value=eye(3)
  Digital Clock : DigitalClock
  Gain : Gain  Gain=1e4
  Magnetic Field Model : Subsystem
  Math Function : Math  Operator=transpose  SaturateOnIntegerOverflow=on
  Math Function1 : Math  Operator=transpose  SaturateOnIntegerOverflow=on
  Matrix Multiply : Product  Multiplication=Matrix(*)
  Matrix Multiply1 : Product  Multiplication=Matrix(*)
  Product : Product  Multiplication=Matrix(*)
  Random Number : RandomNumber  Variance=mag_variance  SampleTime=0.1
  Sine Wave : Sin  Amplitude=0 * 1e-6 * randn(3, 1)  Frequency=2*pi / (90 * 60)  SampleTime=0
  Sum : Sum  Inputs=|++
  Sum1 : Sum  Inputs=|++
  b_S : Outport
  Time : Outport  Port=2
  Magnetometer : Outport  Port=3
  wires:
  Matrix Multiply1/1 -> Sum/1
  Random Number/1 -> Sum/2
  DCM B wrt S/1 -> Math Function/1
  Sum/1 -> Product/2
  Math Function/1 -> Product/1
  Product/1 -> Gain/1
  Gain/1 -> Bus Creator/1, b_S/1
  r_E/1 -> Magnetic Field Model/1(r_E)
  Magnetic Field Model/1(b_E) -> Sum1/1
  Sine Wave/1 -> Sum1/2
  Sum1/1 -> Matrix Multiply/2
  Math Function1/1 -> Matrix Multiply/1
  Matrix Multiply/1 -> Matrix Multiply1/2
  DCM of ECFC wrt ECI/1 -> Math Function1/1
  DCM of BN/1 -> Matrix Multiply1/1
  Digital Clock/1 -> Bus Creator/2, Time/1
  Bus Creator/1 -> Magnetometer/1

== system StateMachinaTesting/Sensors BUSSED/Center Cube Sensors/Subsystem ==
  "a_N " : Inport
  q_BN : Inport  Port=2
  Product : Product  Multiplication=Matrix(*)
  Quaternions to Direction Cosine Matrix : aerolibtransform2/Quaternions to  Direction Cosine Matrix
  a_B : Outport
  wires:
  Quaternions to Direction Cosine Matrix/1 -> Product/1
  Product/1 -> a_B/1
  q_BN/1 -> Quaternions to Direction Cosine Matrix/1
  "a_N "/1 -> Product/2

== system StateMachinaTesting/Sensors BUSSED/Center Cube Sensors/Sun Sensor ==
  In1 : Inport
  Out1 : Outport
  wires:
  In1/1 -> Out1/1

== system StateMachinaTesting/Sensors BUSSED/SideCubeSensors/Create Mag Vector ==
  q_BN : Inport
  r_N : Inport  Port=2
  Constant : Constant  Value=[1 1 1]
  Terminator : Terminator
  Terminator1 : Terminator
  mag_B : Outport
  wires:
  Constant/1 -> mag_B/1
  r_N/1 -> Terminator1/1
  q_BN/1 -> Terminator/1

== system StateMachinaTesting/Sensors BUSSED/SideCubeSensors/Create Sun Vector ==
  q_BN : Inport
  r_N : Inport  Port=2
  time : Inport  Port=3
  Constant1 : Constant  Value=[1 1 1]
  Terminator : Terminator
  Terminator1 : Terminator
  Terminator2 : Terminator
  sun_B : Outport
  wires:
  time/1 -> Terminator2/1
  Constant1/1 -> sun_B/1
  r_N/1 -> Terminator1/1
  q_BN/1 -> Terminator/1

== system StateMachinaTesting/Sensors BUSSED/SideCubeSensors/Frame Convert ==
  a_N : Inport
  q_BN : Inport  Port=2
  Terminator : Terminator
  a_B : Outport
  wires:
  q_BN/1 -> Terminator/1
  a_N/1 -> a_B/1

== system StateMachinaTesting/Sensors BUSSED/SideCubeSensors1/Create Mag Vector ==
  q_BN : Inport
  r_N : Inport  Port=2
  Constant : Constant  Value=[1 1 1]
  Terminator : Terminator
  Terminator1 : Terminator
  mag_B : Outport
  wires:
  Constant/1 -> mag_B/1
  r_N/1 -> Terminator1/1
  q_BN/1 -> Terminator/1

== system StateMachinaTesting/Sensors BUSSED/SideCubeSensors1/Create Sun Vector ==
  q_BN : Inport
  r_N : Inport  Port=2
  time : Inport  Port=3
  Constant1 : Constant  Value=[1 1 1]
  Terminator : Terminator
  Terminator1 : Terminator
  Terminator2 : Terminator
  sun_B : Outport
  wires:
  time/1 -> Terminator2/1
  Constant1/1 -> sun_B/1
  r_N/1 -> Terminator1/1
  q_BN/1 -> Terminator/1

== system StateMachinaTesting/Sensors BUSSED/SideCubeSensors1/Frame Convert ==
  a_N : Inport
  q_BN : Inport  Port=2
  Terminator : Terminator
  a_B : Outport
  wires:
  q_BN/1 -> Terminator/1
  a_N/1 -> a_B/1

== system StateMachinaTesting/Sensors MUXED/Center Cube Sensors/Create Mag Vector ==
  note: r_N is in format:
      | - Lat (N-S) in decimal deg
      | - Long (E-W) in decimal deg
      | - Height in m
  q_BN : Inport
  r_N : Inport  Port=2
  time : Inport  Port=3
  Constant : Constant  Value=1e-9
  Demux : Demux  Outputs=3
  ECI Position to LLA : aerolibtransform2/ECI Position to LLA  red=IAU-2000/2006  year=2016  month=September  day=20  hour=0  min=0  sec=0  deltaT=Sec  errorflag=Error  extraparamflag=off  eunits=Metric (MKS)  earthmodel=WGS84  flat=1/298.257223563  eqradius=6378137
      settings: AttributesFormatString=%<red>
  Product : Product  Multiplication=Matrix(*)
  Product1 : Product
  Quaternions to Direction Cosine Matrix : aerolibtransform2/Quaternions to  Direction Cosine Matrix
  "RBF!!!!! " : Constant  Value=2015
  Terminator{2..5} (4 alike) : Terminator
  World Magnetic Model 2015 : aerolibgravity2/World Magnetic Model 2015  units=Metric (MKS)  time_in=on  month=January  day=1  year=2015  action=Error  h_out=on  dec_out=on  inc_out=on  ti_out=on
  mag_B : Outport
  wires:
  Product/1 -> mag_B/1
  Demux/1 -> World Magnetic Model 2015/2
  Demux/2 -> World Magnetic Model 2015/3
  World Magnetic Model 2015/2 -> Terminator2/1
  World Magnetic Model 2015/3 -> Terminator3/1
  World Magnetic Model 2015/4 -> Terminator4/1
  World Magnetic Model 2015/5 -> Terminator5/1
  time/1 -> ECI Position to LLA/2
  "RBF!!!!! "/1 -> World Magnetic Model 2015/4
  r_N/1 -> ECI Position to LLA/1
  Demux/3 -> World Magnetic Model 2015/1
  ECI Position to LLA/1 -> Demux/1
  q_BN/1 -> Quaternions to Direction Cosine Matrix/1
  Quaternions to Direction Cosine Matrix/1 -> Product/1
  World Magnetic Model 2015/1 -> Product1/2
  Constant/1 -> Product1/1
  Product1/1 -> Product/2

== system StateMachinaTesting/Sensors MUXED/Center Cube Sensors/Create Sun Vector ==
  note: s_hat_N
  note: Outputs the unit vector towards the sun wrt the body (or earth; doesn't matter) in the inertial frame (N).
  q_BN : Inport
  time : Inport  Port=2
  GPS time to Jd sfrom J2000 : Subsystem
  Normalization : dspmathops/Normalization  NormType=2-norm  Bias=1e-10  NormOver=Each column  Dimension=1  outputDataTypeStr=Inherit: Same as product output  outputLastDataTypeStr=Inherit: Same as product output  outputMin=[]  outputMax=[]  accumDataTypeStr=Inherit: Same as product output  accumLastDataTypeStr=Inherit: Same as product output  roundingMode=Floor  overflowMode=off
  Product : Product  Multiplication=Matrix(*)
  Quaternions to Direction Cosine Matrix : aerolibtransform2/Quaternions to  Direction Cosine Matrix
  Sun position off of Jd frm J2000 : Subsystem
  sun_B : Outport
  wires:
  time/1 -> GPS time to Jd sfrom J2000/1(In1)
  Product/1 -> sun_B/1
  q_BN/1 -> Quaternions to Direction Cosine Matrix/1
  Normalization/1 -> Product/2
  Quaternions to Direction Cosine Matrix/1 -> Product/1
  GPS time to Jd sfrom J2000/1(Out1) -> Sun position off of Jd frm J2000/1(In1)
  Sun position off of Jd frm J2000/1(Out1) -> Normalization/1

== system StateMachinaTesting/Sensors MUXED/Center Cube Sensors/Subsystem ==
  "a_N " : Inport
  q_BN : Inport  Port=2
  Product : Product  Multiplication=Matrix(*)
  Quaternions to Direction Cosine Matrix : aerolibtransform2/Quaternions to  Direction Cosine Matrix
  a_B : Outport
  wires:
  Quaternions to Direction Cosine Matrix/1 -> Product/1
  Product/1 -> a_B/1
  q_BN/1 -> Quaternions to Direction Cosine Matrix/1
  "a_N "/1 -> Product/2

== system StateMachinaTesting/x_measured1/Lookup Tables/GPS time to Jd sfrom J2000 ==
  In1 : Inport
  Jd since GPS0 : Constant  Value=2444244.5
  Jd since J2000 : Constant  Value=2451545
  "Leap Seconds from GSP0 " : Constant  Value=27-9
  Sum : Sum  Inputs=|++
  Sum1 : Sum  Inputs=|++
  Sum2 : Sum  Inputs=|+-
  seconds to days conversion : Gain  Gain=1/86400
  Out1 : Outport
  wires:
  Sum2/1 -> Out1/1
  Jd since J2000/1 -> Sum2/2
  Sum1/1 -> Sum2/1
  Jd since GPS0/1 -> Sum1/2
  seconds to days conversion/1 -> Sum1/1
  Sum/1 -> seconds to days conversion/1
  "Leap Seconds from GSP0 "/1 -> Sum/2
  In1/1 -> Sum/1

== system StateMachinaTesting/x_measured1/Lookup Tables/Sun position off of Jd frm J2000 ==
  In1 : Inport
  Gain : Gain  Gain=1.49597871e8
  MATLAB Function : MATLAB Function  TreatAsAtomicUnit=on
  Out1 : Outport
  wires:
  Gain/1 -> Out1/1
  MATLAB Function/1(S_ECI) -> Gain/1
  In1/1 -> MATLAB Function/1(J2000_days)

== system StateMachinaTesting/Flight Controller/Center Cube Controller/Attitude Compensator/Deployed Modes (switch)1 ==
  note: Deployed Block
      | Notes: This block determines the actions the satellite will execute based on the commands given by ground control/ powerboard. The 2 cases are normal operations, and eclipse
  Mode and BurnCmd : Inport
  q1 : Inport  Port=2
  w1 : Inport  Port=3
  Action Port : ActionPort
  Bus Selector : BusSelector  OutputSignals=SafedOpMode,SeperationCommand
  Default : Subsystem  TreatAsAtomicUnit=on
  Deployed : SwitchCase  CaseConditions={7, 12}
  Merge1 : Merge  Inputs=3
  Seek EKF Convergence : Subsystem  TreatAsAtomicUnit=on
  Spin-Up Slew : Subsystem  TreatAsAtomicUnit=on
  Terminator : Terminator
  Out1 : Outport
  wires:
  w1/1 -> Spin-Up Slew/2(w)
  Deployed/1 -> Spin-Up Slew/Action
  Spin-Up Slew/1(tau) -> Merge1/1
  q1/1 -> Spin-Up Slew/1(q)
  Deployed/3 -> Default/Action
  Merge1/1 -> Out1/1
  Mode and BurnCmd/1 -> Bus Selector/1
  Bus Selector/1 -> Deployed/1  "<SafedOpMode>"
  Bus Selector/2 -> Terminator/1  "<SeperationCommand>"
  Default/1(Out1) -> Merge1/3
  Deployed/2 -> Seek EKF Convergence/Action
  Seek EKF Convergence/1(Out1) -> Merge1/2

== system StateMachinaTesting/Flight Controller/Center Cube Controller/Attitude Compensator/Not Deployed Modes (switch) ==
  note: What is the seek EKF Convergence?
  note: Not Deployed Block
      | Notes: This block determines the actions the satellite will execute based on the commands given by ground control/ powerboard. The 3 cases are detumbling, sun pointing, and eclipse
  Mode and BurnCmd : Inport
  q_BN : Inport  Port=2
  w_BN : Inport  Port=3
  Action Port : ActionPort
  Bus Selector : BusSelector  OutputSignals=SafedOpMode,SeperationCommand
  Detumbling Slew : Subsystem  TreatAsAtomicUnit=on
  Inertia : Constant  Value=I_undeployed
  Inital Spin Up : Subsystem  TreatAsAtomicUnit=on
  Merge1 : Merge  Inputs=5
  Not Deployed : SwitchCase  CaseConditions={5,6,7,12}
  Null Case1 : Subsystem  TreatAsAtomicUnit=on
  Seek EKF Convergence : Subsystem  TreatAsAtomicUnit=on
  Sun Pointing : Subsystem  TreatAsAtomicUnit=on
  Terminator : Terminator
  Out1 : Outport
  wires:
  Merge1/1 -> Out1/1
  Not Deployed/5 -> Null Case1/Action
  q_BN/1 -> Sun Pointing/1(q), Inital Spin Up/1(q_BN), Detumbling Slew/1(q_BN)
  Detumbling Slew/1(tau) -> Merge1/1
  Not Deployed/2 -> Sun Pointing/Action
  Sun Pointing/1(tau) -> Merge1/2
  Not Deployed/1 -> Detumbling Slew/Action
  w_BN/1 -> Detumbling Slew/2(w_BN), Sun Pointing/2(w_BN), Inital Spin Up/2(w)
  Mode and BurnCmd/1 -> Bus Selector/1
  Not Deployed/3 -> Inital Spin Up/Action
  Inital Spin Up/1(tau) -> Merge1/3
  Inertia/1 -> Inital Spin Up/3("I "), Detumbling Slew/3("Inertia ")
  Not Deployed/4 -> Seek EKF Convergence/Action
  Null Case1/1(Out1) -> Merge1/5
  Seek EKF Convergence/1(Out1) -> Merge1/4
  Bus Selector/1 -> Not Deployed/1  "<SafedOpMode>"
  Bus Selector/2 -> Terminator/1  "<SeperationCommand>"

== system StateMachinaTesting/Flight Controller/Center Cube Controller/Motor Control Placeholder/Spinning fast ==
  Action Port : ActionPort
  Constant : Constant  Value=0.05
  Out1 : Outport
  wires:
  Constant/1 -> Out1/1

== system StateMachinaTesting/Flight Controller/Center Cube Controller/Motor Control Placeholder/Spinning slow ==
  Action Port : ActionPort
  Constant : Constant  Value=0
  Out1 : Outport
  wires:
  Constant/1 -> Out1/1

== system StateMachinaTesting/Flight Controller/Center Cube Controller/SafeMode/ADCS Subsystem ==
  "ADCSAks " : Inport
  Bus Selector : BusSelector  OutputSignals=SensorsAk,TorquerAk
  Bus Selector1 : BusSelector  OutputSignals=Mag1Ak,Mag2Ak,Accel1Ak,Accel2Ak,Gyro1Ak,Gyro2Ak,SunS1Ak,SunS2Ak
  Bus Selector2 : BusSelector  OutputSignals=TC_X1,TC_Y1,TC_Z1
  Data Type Conversion : DataTypeConversion
  IMU : Subsystem
  Logical Operator1 : Logic  Operator=OR  AllPortsSameDT=off  OutDataTypeStr=boolean
  Magnetic Torquers : Subsystem
  Mux : Mux
  Mux1 : Mux  Inputs=3
  Mux3 : Mux  Inputs=3
  Mux4 : Mux  Inputs=2
  Mux5 : Mux  Inputs=2
  "ADCSs " : Outport
  wires:
  Bus Selector2/3 -> Magnetic Torquers/3(Magnetometer Z1)  "<TC_Z1>"
  Bus Selector2/2 -> Magnetic Torquers/2(Magnetometer Y1)  "<TC_Y1>"
  Mux1/1 -> "ADCSs "/1  "ADCS Health"
  Mux4/1 -> Mux1/2  "ADCS Sectional Status"
  IMU/1(Magnetometer) -> Mux/1  "Magnetometer Health"
  IMU/3(Accelerometer) -> Mux/3  "Accelerometer Health"
  IMU/2("Gyro ") -> Mux/2  "Gyro Health"
  IMU/5(IMU Health) -> Mux4/1, Logical Operator1/1  "IMU Health"
  Magnetic Torquers/2("Y Torquer Status ") -> Mux3/2  "Y Torquer Status"
  Magnetic Torquers/1(X Torquer Status) -> Mux3/1  "X Torquer Status"
  Bus Selector2/1 -> Magnetic Torquers/1(Magnetorquer X1)  "<TC_X1>"
  IMU/4("Sun Sensor ") -> Mux/4  "Sun Sensor"
  Logical Operator1/1 -> Mux1/1  "ADCS Functional Status"
  Mux5/1 -> Mux1/3  "ADCS Component Status"
  Mux3/1 -> Data Type Conversion/1  "Torquer Status Array"
  Magnetic Torquers/4(Actuator Health) -> Mux4/2, Logical Operator1/2  "Actuator Health"
  Mux/1 -> Mux5/1  "Sensor Status Array"
  Magnetic Torquers/3(Z Torquer Status) -> Mux3/3  "Z Torquer Status"
  "ADCSAks "/1 -> Bus Selector/1
  Bus Selector/2 -> Bus Selector2/1  "<TorquerAk>"
  Bus Selector/1 -> Bus Selector1/1  "<SensorsAk>"
  Bus Selector1/1 -> IMU/1(Magnetometer 1)  "<Mag1Ak>"
  Bus Selector1/2 -> IMU/2(Magnetometer 2)  "<Mag2Ak>"
  Bus Selector1/3 -> IMU/3(Accelerometer 1)  "<Accel1Ak>"
  Bus Selector1/4 -> IMU/4(" Accelerometer 2")  "<Accel2Ak>"
  Bus Selector1/5 -> IMU/5(Gyro 1)  "<Gyro1Ak>"
  Bus Selector1/6 -> IMU/6(Gyro 2)  "<Gyro2Ak>"
  Bus Selector1/7 -> IMU/7(Sun Sensor 1)  "<SunS1Ak>"
  Bus Selector1/8 -> IMU/8(Sun Sensor 2)  "<SunS2Ak>"
  Data Type Conversion/1 -> Mux5/2

== system StateMachinaTesting/Flight Controller/Center Cube Controller/Torque Coil Management/Measurement Predicition ==
  note: Predicitoon Block
      | This block takes in the current time and the expected time when the action will be executed in order to give a better predicition of what the attitude of the satellite will be at.
  GPS_time : Inport
  something else : Inport  Port=2
  Constant : Constant
  Terminator : Terminator
  Terminator1 : Terminator
  predicition : Outport
  wires:
  GPS_time/1 -> Terminator/1
  something else/1 -> Terminator1/1
  Constant/1 -> predicition/1

== system StateMachinaTesting/Flight Controller/Center Cube Controller/Torque Coil Management/No Action ==
  Action Port : ActionPort
  Constant : Constant  Value=[ 0 0 0 ]
  Constant2 : Constant  Value=[ 0 0 0 ]
  I_coils : Outport
  torque_coils : Outport  Port=2
  wires:
  Constant/1 -> I_coils/1
  Constant2/1 -> torque_coils/1

== system StateMachinaTesting/Flight Controller/Center Cube Controller/Torque Coil Management/PD Controller ==
  note: Controller
      | At this moment in time, I am not sure what this block does, but it appears to be a PD controller with feedforward control that outputs the torque the coils are required to exert. In short, a simple/not-simple controller
  In1 : Inport
  torque_coils : Outport
  wires:
  In1/1 -> torque_coils/1
